simulink model "TestTustin"  (R2022a)
settings: Solver=VariableStepAuto  StartTime=0.0  StopTime=20.0  RelTol=1e-3
settings Model: Creator=paolo  LastModifiedBy=paolo

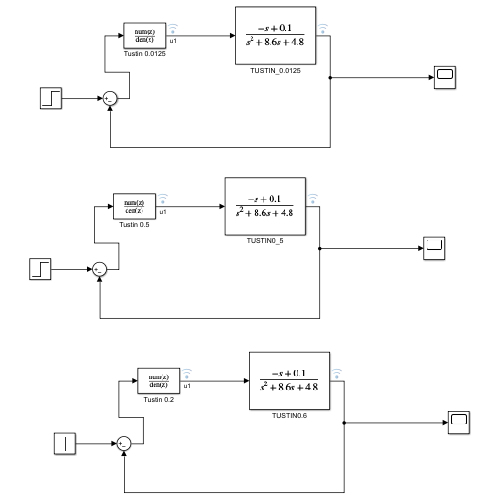
[thumbnail: Simulink's stored preview of the top-level diagram]
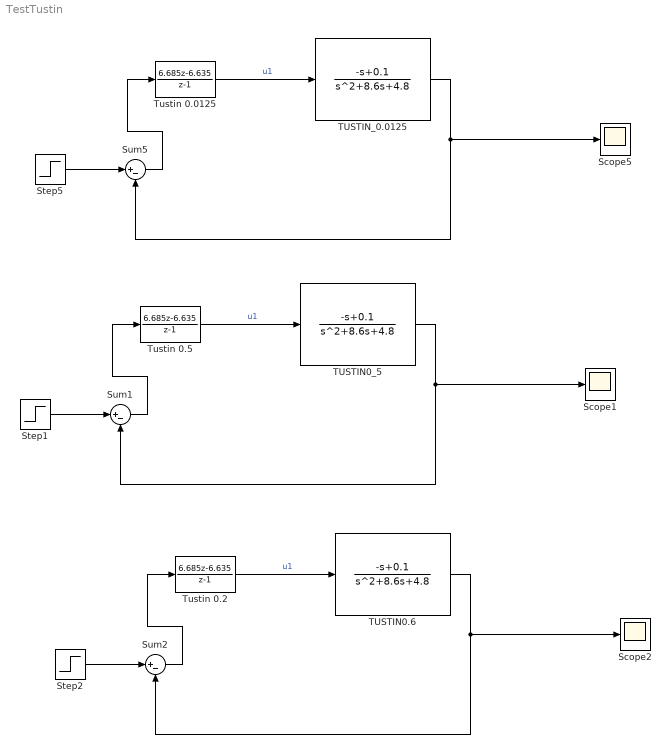
== system TestTustin ==
  Scope1 : Scope
  Scope2 : Scope
  Scope5 : Scope
  Step1 : Step  Time=0  SampleTime=0
  Step2 : Step  Time=0  SampleTime=0
  Step5 : Step  Time=0  SampleTime=0
  Sum1 : Sum  Inputs=|+-
  Sum2 : Sum  Inputs=|+-
  Sum5 : Sum  Inputs=|+-
  TUSTIN0.6 : TransferFcn  Numerator=[-1, 0.1]  Denominator=[1, 8.6, 4.8]
  TUSTIN0_5 : TransferFcn  Numerator=[-1, 0.1]  Denominator=[1, 8.6, 4.8]
  TUSTIN_0.0125 : TransferFcn  Numerator=[-1, 0.1]  Denominator=[1, 8.6, 4.8]
  Tustin 0.0125 : DiscreteTransferFcn  Numerator=[6.685, -6.635]  Denominator=[1, -1]  SampleTime=0.0125
  Tustin 0.2 : DiscreteTransferFcn  Numerator=[6.685, -6.635]  Denominator=[1, -1]  SampleTime=0.6
  Tustin 0.5 : DiscreteTransferFcn  Numerator=[6.685, -6.635]  Denominator=[1, -1]  SampleTime=0.5
  wires:
  Tustin 0.0125/1 -> TUSTIN_0.0125/1  "u1"
  Sum5/1 -> Tustin 0.0125/1
  Step5/1 -> Sum5/1
  TUSTIN_0.0125/1 -> Sum5/2, Scope5/1
  Tustin 0.5/1 -> TUSTIN0_5/1  "u1"
  TUSTIN0_5/1 -> Sum1/2, Scope1/1
  Step1/1 -> Sum1/1
  Sum1/1 -> Tustin 0.5/1
  Tustin 0.2/1 -> TUSTIN0.6/1  "u1"
  TUSTIN0.6/1 -> Sum2/2, Scope2/1
  Step2/1 -> Sum2/1
  Sum2/1 -> Tustin 0.2/1
